simulink model "exp11"  (R2025b)
settings: Solver=VariableStepAuto  StartTime=0.0  StopTime=10.0  RelTol=1e-3
settings Model: Creator=shanm  LastModifiedBy=SUBHASH

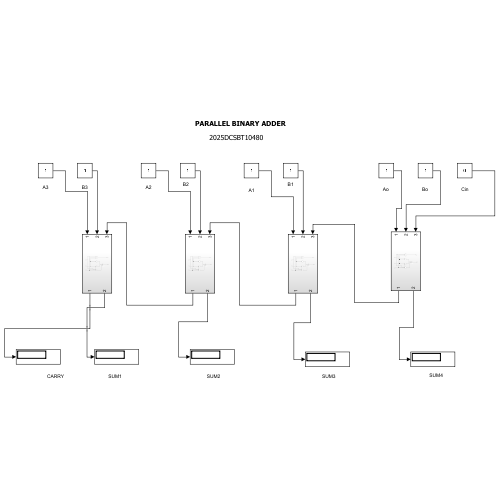
[thumbnail: Simulink's stored preview of the top-level diagram]
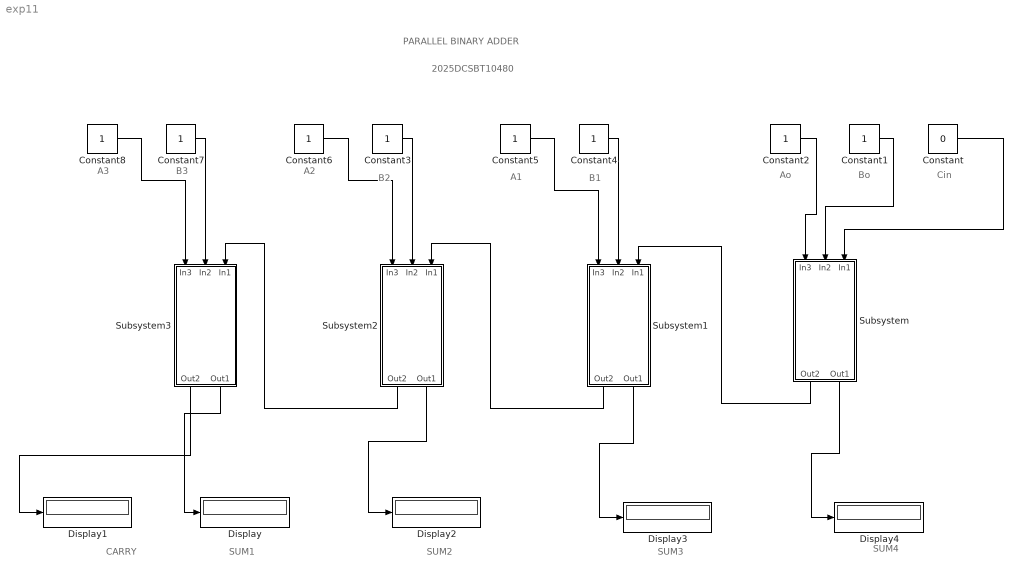
== system exp11 ==
  note: 2025DCSBT10480
  note: Cin
  note: CARRY
  note: SUM1
  note: SUM2
  note: SUM3
  note: SUM4
  note: Bo
  note: Ao
  note: B1
  note: A1
  note: B2
  note: A2
  note: B3
  note: A3
  note: PARALLEL BINARY ADDER
  Constant : Constant  Value=0
  Constant{1..8} (8 alike) : Constant
  Display{,1..4} (5 alike) : Display
  Subsystem : Subsystem
      settings: PortSchema="{\"entries\":[{\"content\":{\"sides\":[{\"content\":{},\"type\":\"ConnectorPlacement.EquallySpacedRectSide\",\"uuid\":\"108d892a-8720-40a2-8c7e-3ae5f46a708e\"},{\"content\":{\"side\":\"RIGHT\"},\"type\":\"ConnectorPlacement.EquallySpacedRectSide\",\"uuid\":\"3570579f-a2bf-462b-b3db-0cdd64646b39\"},{\"content\":{\"connectorIds\":[\"In1\",\"In2\",\"In3\"],\"side\":\"TOP\"},\"type\":\"ConnectorPlacement.EquallySpacedRectSide\",\"uuid\":\"4551d649-7472-4003-a88b-0ff586cc678a\"},{\"content\":{\"connectorIds\":[\"Out1\",\"Out2\"],\"side\":\"BOTTOM\"},\"type\":\"ConnectorPlacement.EquallySpacedRectSide\",\"uuid\":\"a5f06a54-db33-4349-ad01-48478af09889\"}]},\"type\":\"ConnectorPlacement.EquallySpacedConnector\",\"uuid\":\"0c68deb8-0e0b-4618-934f-8c534f6b83f5\"}],\"packageUris\":[\"http://schema.mathworks.com/mf0/Connector/R2020b\"],\"version\":\"1.0\"}"
  Subsystem1 : Subsystem
      settings: PortSchema="{\"entries\":[{\"content\":{\"sides\":[{\"content\":{},\"type\":\"ConnectorPlacement.EquallySpacedRectSide\",\"uuid\":\"108d892a-8720-40a2-8c7e-3ae5f46a708e\"},{\"content\":{\"side\":\"RIGHT\"},\"type\":\"ConnectorPlacement.EquallySpacedRectSide\",\"uuid\":\"3570579f-a2bf-462b-b3db-0cdd64646b39\"},{\"content\":{\"connectorIds\":[\"In1\",\"In2\",\"In3\"],\"side\":\"TOP\"},\"type\":\"ConnectorPlacement.EquallySpacedRectSide\",\"uuid\":\"4551d649-7472-4003-a88b-0ff586cc678a\"},{\"content\":{\"connectorIds\":[\"Out1\",\"Out2\"],\"side\":\"BOTTOM\"},\"type\":\"ConnectorPlacement.EquallySpacedRectSide\",\"uuid\":\"a5f06a54-db33-4349-ad01-48478af09889\"}]},\"type\":\"ConnectorPlacement.EquallySpacedConnector\",\"uuid\":\"0c68deb8-0e0b-4618-934f-8c534f6b83f5\"}],\"packageUris\":[\"http://schema.mathworks.com/mf0/Connector/R2020b\"],\"version\":\"1.0\"}"
  Subsystem2 : Subsystem
      settings: PortSchema="{\"entries\":[{\"content\":{\"sides\":[{\"content\":{},\"type\":\"ConnectorPlacement.EquallySpacedRectSide\",\"uuid\":\"108d892a-8720-40a2-8c7e-3ae5f46a708e\"},{\"content\":{\"side\":\"RIGHT\"},\"type\":\"ConnectorPlacement.EquallySpacedRectSide\",\"uuid\":\"3570579f-a2bf-462b-b3db-0cdd64646b39\"},{\"content\":{\"connectorIds\":[\"In1\",\"In2\",\"In3\"],\"side\":\"TOP\"},\"type\":\"ConnectorPlacement.EquallySpacedRectSide\",\"uuid\":\"4551d649-7472-4003-a88b-0ff586cc678a\"},{\"content\":{\"connectorIds\":[\"Out1\",\"Out2\"],\"side\":\"BOTTOM\"},\"type\":\"ConnectorPlacement.EquallySpacedRectSide\",\"uuid\":\"a5f06a54-db33-4349-ad01-48478af09889\"}]},\"type\":\"ConnectorPlacement.EquallySpacedConnector\",\"uuid\":\"0c68deb8-0e0b-4618-934f-8c534f6b83f5\"}],\"packageUris\":[\"http://schema.mathworks.com/mf0/Connector/R2020b\"],\"version\":\"1.0\"}"
  Subsystem3 : Subsystem
      settings: PortSchema="{\"entries\":[{\"content\":{\"sides\":[{\"content\":{},\"type\":\"ConnectorPlacement.EquallySpacedRectSide\",\"uuid\":\"108d892a-8720-40a2-8c7e-3ae5f46a708e\"},{\"content\":{\"side\":\"RIGHT\"},\"type\":\"ConnectorPlacement.EquallySpacedRectSide\",\"uuid\":\"3570579f-a2bf-462b-b3db-0cdd64646b39\"},{\"content\":{\"connectorIds\":[\"In1\",\"In2\",\"In3\"],\"side\":\"TOP\"},\"type\":\"ConnectorPlacement.EquallySpacedRectSide\",\"uuid\":\"4551d649-7472-4003-a88b-0ff586cc678a\"},{\"content\":{\"connectorIds\":[\"Out1\",\"Out2\"],\"side\":\"BOTTOM\"},\"type\":\"ConnectorPlacement.EquallySpacedRectSide\",\"uuid\":\"a5f06a54-db33-4349-ad01-48478af09889\"}]},\"type\":\"ConnectorPlacement.EquallySpacedConnector\",\"uuid\":\"0c68deb8-0e0b-4618-934f-8c534f6b83f5\"}],\"packageUris\":[\"http://schema.mathworks.com/mf0/Connector/R2020b\"],\"version\":\"1.0\"}"
  wires:
  Constant/1 -> Subsystem/3(In1)
  Constant1/1 -> Subsystem/2(In2)
  Constant2/1 -> Subsystem/1(In3)
  Constant5/1 -> Subsystem1/1(In3)
  Constant4/1 -> Subsystem1/2(In2)
  Constant6/1 -> Subsystem2/1(In3)
  Constant3/1 -> Subsystem2/2(In2)
  Constant8/1 -> Subsystem3/1(In3)
  Constant7/1 -> Subsystem3/2(In2)
  Subsystem/1(Out2) -> Subsystem1/3(In1)
  Subsystem/2(Out1) -> Display4/1
  Subsystem1/2(Out1) -> Display3/1
  Subsystem1/1(Out2) -> Subsystem2/3(In1)
  Subsystem2/2(Out1) -> Display2/1
  Subsystem2/1(Out2) -> Subsystem3/3(In1)
  Subsystem3/1(Out2) -> Display1/1
  Subsystem3/2(Out1) -> Display/1

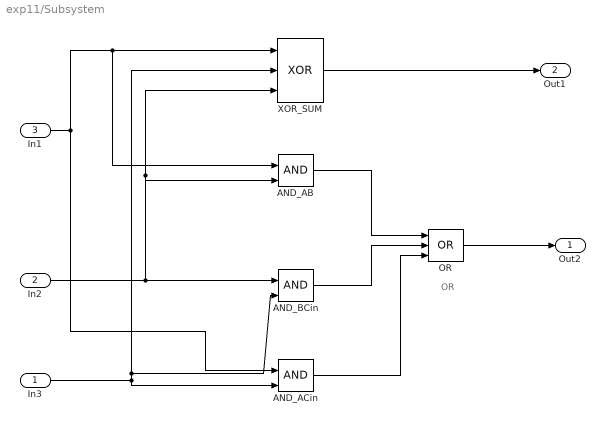
== system exp11/Subsystem ==
  note: OR
  In3 : Inport
  In2 : Inport  Port=2
  In1 : Inport  Port=3
  "AND_AB " : Logic  IconShape=distinctive  AllPortsSameDT=off  OutDataTypeStr=boolean
  AND_ACin : Logic  IconShape=distinctive  AllPortsSameDT=off  OutDataTypeStr=boolean
  AND_BCin : Logic  IconShape=distinctive  AllPortsSameDT=off  OutDataTypeStr=boolean
  OR : Logic  Operator=OR  Inputs=3  IconShape=distinctive  AllPortsSameDT=off  OutDataTypeStr=boolean
  XOR_SUM : Logic  Operator=XOR  Inputs=3  IconShape=distinctive  AllPortsSameDT=off  OutDataTypeStr=boolean
  Out2 : Outport
  Out1 : Outport  Port=2
  wires:
  AND_ACin/1 -> OR/3
  In3/1 -> XOR_SUM/2, AND_BCin/2, AND_ACin/2
  "AND_AB "/1 -> OR/1
  In1/1 -> "AND_AB "/1, XOR_SUM/1, AND_ACin/1
  AND_BCin/1 -> OR/2
  In2/1 -> "AND_AB "/2, XOR_SUM/3, AND_BCin/1
  XOR_SUM/1 -> Out1/1
  OR/1 -> Out2/1

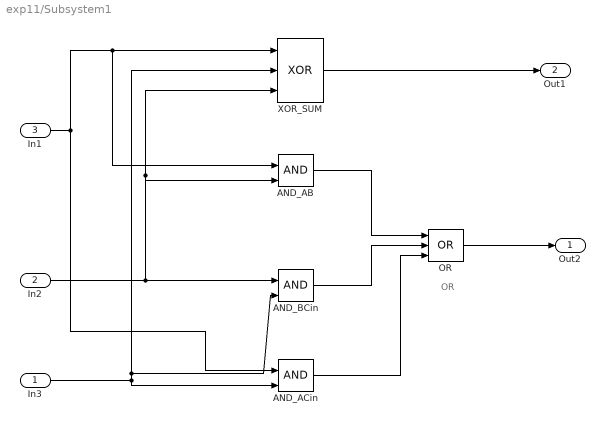
== system exp11/Subsystem1 ==
  note: OR
  In3 : Inport
  In2 : Inport  Port=2
  In1 : Inport  Port=3
  "AND_AB " : Logic  IconShape=distinctive  AllPortsSameDT=off  OutDataTypeStr=boolean
  AND_ACin : Logic  IconShape=distinctive  AllPortsSameDT=off  OutDataTypeStr=boolean
  AND_BCin : Logic  IconShape=distinctive  AllPortsSameDT=off  OutDataTypeStr=boolean
  OR : Logic  Operator=OR  Inputs=3  IconShape=distinctive  AllPortsSameDT=off  OutDataTypeStr=boolean
  XOR_SUM : Logic  Operator=XOR  Inputs=3  IconShape=distinctive  AllPortsSameDT=off  OutDataTypeStr=boolean
  Out2 : Outport
  Out1 : Outport  Port=2
  wires:
  AND_ACin/1 -> OR/3
  In3/1 -> XOR_SUM/2, AND_BCin/2, AND_ACin/2
  "AND_AB "/1 -> OR/1
  In1/1 -> "AND_AB "/1, XOR_SUM/1, AND_ACin/1
  AND_BCin/1 -> OR/2
  In2/1 -> "AND_AB "/2, XOR_SUM/3, AND_BCin/1
  XOR_SUM/1 -> Out1/1
  OR/1 -> Out2/1

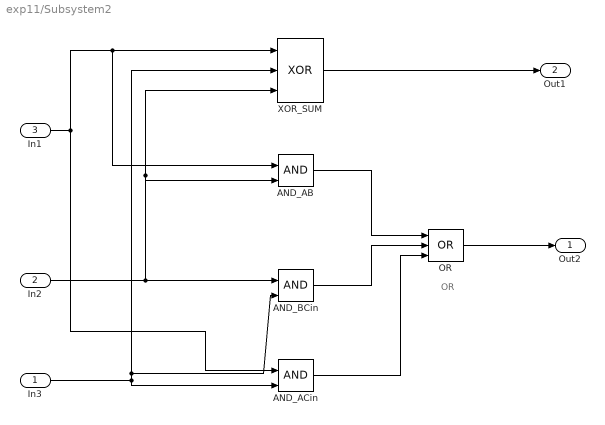
== system exp11/Subsystem2 ==
  note: OR
  In3 : Inport
  In2 : Inport  Port=2
  In1 : Inport  Port=3
  "AND_AB " : Logic  IconShape=distinctive  AllPortsSameDT=off  OutDataTypeStr=boolean
  AND_ACin : Logic  IconShape=distinctive  AllPortsSameDT=off  OutDataTypeStr=boolean
  AND_BCin : Logic  IconShape=distinctive  AllPortsSameDT=off  OutDataTypeStr=boolean
  OR : Logic  Operator=OR  Inputs=3  IconShape=distinctive  AllPortsSameDT=off  OutDataTypeStr=boolean
  XOR_SUM : Logic  Operator=XOR  Inputs=3  IconShape=distinctive  AllPortsSameDT=off  OutDataTypeStr=boolean
  Out2 : Outport
  Out1 : Outport  Port=2
  wires:
  AND_ACin/1 -> OR/3
  In3/1 -> XOR_SUM/2, AND_BCin/2, AND_ACin/2
  "AND_AB "/1 -> OR/1
  In1/1 -> "AND_AB "/1, XOR_SUM/1, AND_ACin/1
  AND_BCin/1 -> OR/2
  In2/1 -> "AND_AB "/2, XOR_SUM/3, AND_BCin/1
  XOR_SUM/1 -> Out1/1
  OR/1 -> Out2/1

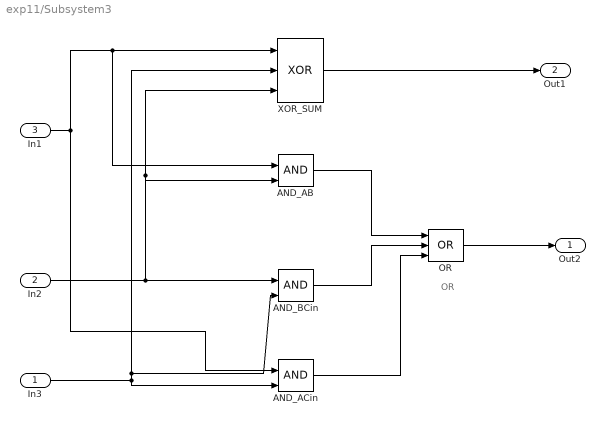
== system exp11/Subsystem3 ==
  note: OR
  In3 : Inport
  In2 : Inport  Port=2
  In1 : Inport  Port=3
  "AND_AB " : Logic  IconShape=distinctive  AllPortsSameDT=off  OutDataTypeStr=boolean
  AND_ACin : Logic  IconShape=distinctive  AllPortsSameDT=off  OutDataTypeStr=boolean
  AND_BCin : Logic  IconShape=distinctive  AllPortsSameDT=off  OutDataTypeStr=boolean
  OR : Logic  Operator=OR  Inputs=3  IconShape=distinctive  AllPortsSameDT=off  OutDataTypeStr=boolean
  XOR_SUM : Logic  Operator=XOR  Inputs=3  IconShape=distinctive  AllPortsSameDT=off  OutDataTypeStr=boolean
  Out2 : Outport
  Out1 : Outport  Port=2
  wires:
  AND_ACin/1 -> OR/3
  In3/1 -> XOR_SUM/2, AND_BCin/2, AND_ACin/2
  "AND_AB "/1 -> OR/1
  In1/1 -> "AND_AB "/1, XOR_SUM/1, AND_ACin/1
  AND_BCin/1 -> OR/2
  In2/1 -> "AND_AB "/2, XOR_SUM/3, AND_BCin/1
  XOR_SUM/1 -> Out1/1
  OR/1 -> Out2/1
